simulink model "dspsrcnv"  (Simulink 6.0)
settings: Solver=FixedStepDiscrete  SolverMode=SingleTasking  StartTime=0.0  StopTime=99.0  RelTol=1e-3  AbsTol=1e-6
libraries: dspsigops x3, dspbuff3 x2, dsparch4 x1, dspmlti3 x1, dspsrcs4 x1
settings Model: RequirementInfo=9  CovMetricSettings=d  Creator=edecosta  LastModifiedBy=sconahan  ExtModeTrigMode=oneshot  ExtModeArmWhenConnect=off
settings DataIOCC: LimitDataPoints=off  SaveOutput=off  SaveTime=off  SignalLoggingName=sigsOut
settings OptimizationCC: BlockReduction=off  BooleanDataType=off  MultiInstanced=off  RollThreshold=2
settings FormatCC: IgnoreBidirectionalLines=off
settings DebuggingCC: IntegerOverflowMsg=none
settings HardwareCC: TargetUnknown=on
settings CodeAppCC: FileBanners=off  CustomSymbols=off
settings GRTTargetCC: TargetFcnLib=iso_c_tmw.mat  IsERTTarget=off

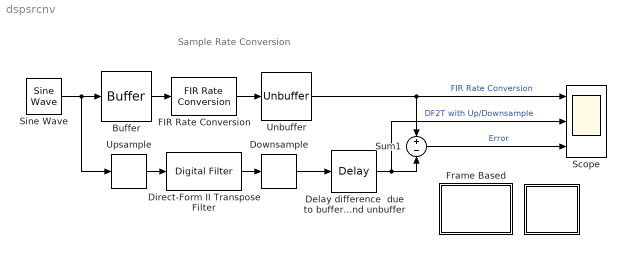
== system dspsrcnv ==
  note: Sample Rate Conversion
  " " : Subsystem
      mask Display: disp('Info')
  Buffer : dspbuff3/Buffer  N=5  V=0  ic=0
  Delay difference  due to buffer  and unbuffer : dspsigops/Delay  dly_unit=Samples  delay=39  ic_detail=on  dif_ic_for_ch=off  dif_ic_for_dly=off  ic=0  reset_popup=None
  Direct-Form II Transpose Filter : dsparch4/Digital Filter  TypePopup=FIR (all zeros)  IIRFiltStruct=Direct form II transposed  AllPoleFiltStruct=Direct form  FIRFiltStruct=Direct form  CoeffSource=Specify via dialog  NumCoeffs=fir1(63,1/8)*8  DenCoeffs=[1 0.1]  BiQuadCoeffs=[1 0.3 0.4 1 0.1 0.2]  LatticeCoeffs=[0.2 0.4]  denIgnore=on  FiltPerSampPopup=One filter per frame  IC=0  ICnum=0  ICden=0  roundingMode=Floor  overflowMode=off
  Downsample : dspsigops/Downsample  N=5  phase=0  ic=0  smode=Allow multirate  fmode=Maintain input frame size
  FIR Rate Conversion : dspmlti3/FIR Rate Conversion  L=8  h=fir1(63,1/8)*8  M=5  roundingMode=Floor  overflowMode=off
  Frame Based : Subsystem
      settings: OpenFcn=dspsrcnvf;
      mask Display: disp('Frame-based\nVersion')
  Scope : Scope  NumInputPorts=3
      settings: TimeRange=99  YMin=-1.1~-1.1~-0.0120167  YMax=1.1~1.1~0.0127305
  Sine Wave : dspsrcs4/Sine Wave  Amplitude=1  Frequency=0.1  Phase=0  SampleMode=Discrete  OutComplex=Real  CompMethod=Trigonometric fcn  TableSize=Speed  SampleTime=1  SamplesPerFrame=1  dataType=double  wordLen=16  udDataType=sfix(16)  fracBitsMode=Best precision  numFracBits=14  ResetState=Restart at time zero
  Sum1 : Sum  Inputs=+-  SaturateOnIntegerOverflow=on  InputSameDT=on
  Unbuffer : dspbuff3/Unbuffer  ic=0
  Upsample : dspsigops/Upsample  N=8  phase=5  ic=0  mode=Maintain input frame size
  wires:
  Sine Wave/1 -> Buffer/1, Upsample/1
  FIR Rate Conversion/1 -> Unbuffer/1
  Buffer/1 -> FIR Rate Conversion/1
  Direct-Form II Transpose Filter/1 -> Downsample/1
  Upsample/1 -> Direct-Form II Transpose Filter/1
  Downsample/1 -> Delay difference  due to buffer  and unbuffer/1
  Unbuffer/1 -> Sum1/1, Scope/1  "FIR Rate Conversion"
  Delay difference  due to buffer  and unbuffer/1 -> Sum1/2, Scope/2  "DF2T with Up/Downsample"
  Sum1/1 -> Scope/3  "Error"

== system dspsrcnv/  ==
  note: Digital Sample Rate Conversion:
      |   Sample-Based Implementation
  note: The filter is used to bandlimit the signal to 1/max(M,L), where M and L
      | are the downsampling and upsampling factors, respectively.
      | Filter order should be sufficiently high so as to yield satisfactory
      | reduction of aliasing and imaging artifacts.
      |
      | Compare the execution speed of this demo vs. that of
      | the frame-based implementation.
  note: This system demonstrates the equivalence between the "FIR
      | Rate Conversion"  block and the straightforward but far less
      | efficient system consisting of separate upsampling, FIR filtering,
      | and downsampling blocks.  Note that there is a delay
      | between the input signal and the rate-conversion result.
      |
      | Efficiency is gained by employing a polyphase implementation
      | for up- and down-sampling.  This technique effectively eliminates
      | all multiplication by zeros (during the interpolation process) and
      | computation of discarded outputs (during the decimation process).
      |
      | The rate conversion must be chosen to be a ratio of relatively
      | prime integers, such as 8/5 as in the example.  An arbitrary
      | integer ratio may be easily converted to a relatively prime ratio
      | by dividing by the GCD (greatest common divisor).

== system dspsrcnv/Frame Based ==
